simulink model "full_system_boat"  (R2025b)
settings: Solver=FixedStepAuto  StartTime=0.0  StopTime=90  RelTol=1e-3  EnableMultiTasking=on
libraries: arduinolib x7, arduinowifilib x6, dspnetwork x3
settings Model: ExtModeTrigDuration=2  Creator=M  LastModifiedBy=M
settings SolverCC: AutoInsertRateTranBlk=on
settings OptimizationCC: EnhancedBackFolding=on  PassReuseOutputArgsAs=Individual arguments  ZeroExternalMemoryAtStartup=off  ZeroInternalMemoryAtStartup=off  MaxStackSize=64  OptimizeBlockOrder=speed  DifferentSizesBufferReuse=on  OptimizationCustomize=off  EfficientTunableParamExpr=on
settings DebuggingCC: ParameterTunabilityLossMsg=error
settings HardwareCC: ProdBitPerPointer=32.0  ProdBitPerSizeT=32.0  ProdBitPerPtrDiffT=32.0  ProdLargestAtomicInteger=Long  ProdLargestAtomicFloat=Double  ProdWordSize=32.0  ProdHWDeviceType=ARM Compatible->ARM Cortex  UseEmbeddedCoderFeatures=off  UseSimulinkCoderFeatures=off
settings SFSimCC: MATLABDynamicMemAlloc=off
settings RTWCC: SystemTargetFile=ert.tlc  HardwareBoard=ESP32-WROOM (Arduino Compatible)  TLCOptions="-aInlineSetEventsForThisBaseRateFcn=TLC_FALSE -aSuppressMultiTaskScheduler=TLC_FALSE  -aRateBasedStepFcn=0"  TemplateMakefile=ert_default_tmf  Toolchain=ESP32  BuildConfiguration=Faster Runs  Description=Embedded Coder
settings CodeAppCC: ForceParamTrailComments=on  IgnoreCustomStorageClasses=off  OperatorAnnotations=on  SimulinkDataObjDesc=on  SFDataObjDesc=on  MangleLength=10.0  InsertBlockDesc=on
settings ERTTargetCC: ExtModeTransport=3.0  ExtModeStaticAlloc=on  ExtModeAutomaticAllocSize=off  ExtModeStaticAllocSize=65536.0  ExtModeMexFile=ext_xcp  ExtModeIntrfLevel=Level2 - Open  InlinedParameterPlacement=Hierarchical  SupportContinuousTime=on  SupportNonInlinedSFcns=on  SupportVariableSizeSignals=on

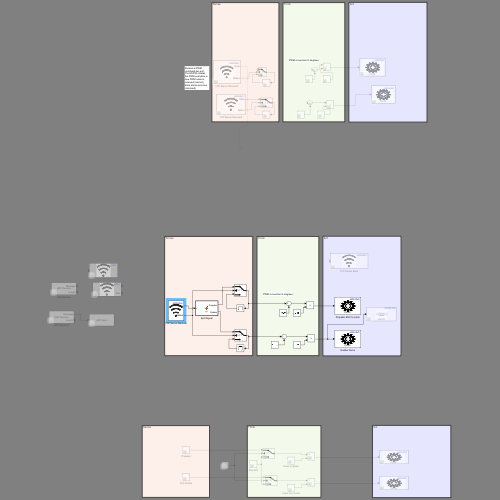
[thumbnail: Simulink's stored preview of the top-level diagram]
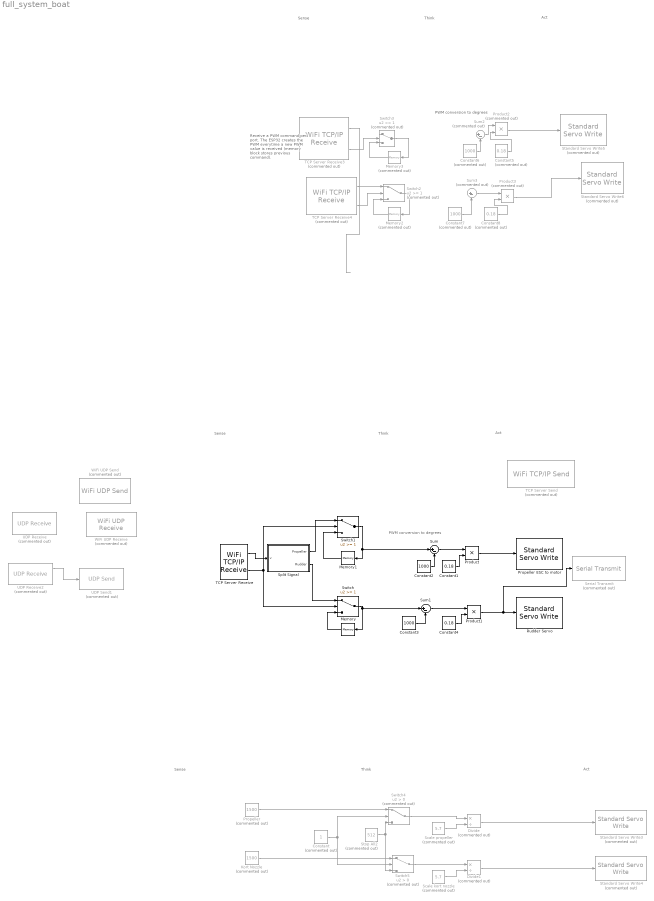
== system full_system_boat ==
  note: Think
  note: PWM conversion to degrees
  note: Sense
  note: Act
  note: Sense
  note: Think
  note: Act
  note: Sense
  note: Receive a PWM command per port. The ESP32 creates the PWM everytime a new PWM value is received (memory block stores previous command).
  note: Act
  note: PWM conversion to degrees
  note: Think
  Constant : Constant  Commented=on  OutDataTypeStr=double
  Constant1 : Constant  Value=0.18  OutDataTypeStr=single
  Constant2 : Constant  Value=1000  OutDataTypeStr=single
  Constant3 : Constant  Value=1000  OutDataTypeStr=single
  Constant4 : Constant  Value=0.18  OutDataTypeStr=single
  Constant5 : Constant  Commented=on  Value=0.18  OutDataTypeStr=single
  Constant6 : Constant  Commented=on  Value=1000  OutDataTypeStr=single
  Constant7 : Constant  Commented=on  Value=1000  OutDataTypeStr=single
  Constant8 : Constant  Commented=on  Value=0.18  OutDataTypeStr=single
  Divide : Product  Commented=on  Inputs=*/
  Divide1 : Product  Commented=on  Inputs=*/
  Kort Nozzle : Constant  Commented=on  Value=1500  OutDataTypeStr=double
  Memory : Memory  InitialCondition=1500
  Memory1 : Memory  InitialCondition=1500
  Memory2 : Memory  Commented=on  InitialCondition=1500
  Memory3 : Memory  Commented=on  InitialCondition=1500
  Product : Product  OutDataTypeStr=single  RndMeth=Nearest
  Product1 : Product  OutDataTypeStr=single  RndMeth=Nearest
  Product2 : Product  Commented=on  OutDataTypeStr=single  RndMeth=Nearest
  Product3 : Product  Commented=on  OutDataTypeStr=single  RndMeth=Nearest
  Propeller : Constant  Commented=on  Value=1500  OutDataTypeStr=double
  Propeller ESC to motor : arduinolib/Standard Servo Write  pinNumber=26  ServoIndex=0  blockPlatform=ESP32
  Rudder Servo : arduinolib/Standard Servo Write  pinNumber=25  ServoIndex=1  blockPlatform=ESP32
  Scale kort nozzle : Constant  Commented=on  Value=5.7
  Scale propeller : Constant  Commented=on  Value=5.7
  Serial Transmit : arduinolib/Serial Transmit  Commented=on  portNumber=0  sendmode=println  label=prop=  sendformat=Decimal  floatprecision=1  header=[]  terminator=[]  blockPlatform=ARDUINO
  Split Signal : MATLAB Function  TreatAsAtomicUnit=on
  Standard Servo Write3 : arduinolib/Standard Servo Write  Commented=on  pinNumber=26  ServoIndex=0  blockPlatform=ESP32
  Standard Servo Write4 : arduinolib/Standard Servo Write  Commented=on  pinNumber=25  ServoIndex=1  blockPlatform=ESP32
  Standard Servo Write5 : arduinolib/Standard Servo Write  Commented=on  pinNumber=26  ServoIndex=0  blockPlatform=ESP32
  Standard Servo Write6 : arduinolib/Standard Servo Write  Commented=on  pinNumber=25  ServoIndex=0  blockPlatform=ESP32
  Stop All2 : Constant  Commented=on  Value=512  OutDataTypeStr=double
  Sum : Sum  Inputs=|+-  OutDataTypeStr=single  RndMeth=Nearest
  Sum1 : Sum  Inputs=|+-  OutDataTypeStr=single  RndMeth=Nearest
  Sum2 : Sum  Commented=on  Inputs=|+-  OutDataTypeStr=single  RndMeth=Nearest
  Sum3 : Sum  Commented=on  Inputs=|+-  OutDataTypeStr=single  RndMeth=Nearest
  Switch : Switch  Threshold=1  RndMeth=Nearest  SaturateOnIntegerOverflow=off  InputSameDT=off
  Switch1 : Switch  Threshold=1  RndMeth=Nearest  SaturateOnIntegerOverflow=off  InputSameDT=off
  Switch2 : Switch  Commented=on  Threshold=1  RndMeth=Nearest  SaturateOnIntegerOverflow=off  InputSameDT=off
  Switch3 : Switch  Commented=on  Threshold=1  RndMeth=Nearest  SaturateOnIntegerOverflow=off  InputSameDT=off
  Switch4 : Switch  Commented=on  Criteria=u2 > Threshold  RndMeth=Nearest  SaturateOnIntegerOverflow=off  InputSameDT=off
  Switch5 : Switch  Commented=on  Criteria=u2 > Threshold  SaturateOnIntegerOverflow=off  InputSameDT=off
  TCP Server Receive : arduinowifilib/WiFi TCP//IP Receive  Mode_=Server  serverport=2000  RemoteAddr_=192.168.137.1  RemoteServerPort_=10000  DataType_=single  DataSize_=2  SampleTime_=0.02  remoteipoctet1=192  remoteipoctet2=168  remoteipoctet3=137  remoteipoctet4=1  wifiTCPServerIndex=0  wifiTCPClientIndex=0  blockPlatform=ARDUINO  isARMArch=false  BlockingMode_=off  BlockTimeout_=0.03
  TCP Server Receive3 : arduinowifilib/WiFi TCP//IP Receive  Commented=on  Mode_=Server  serverport=20001  RemoteAddr_=192.168.137.1  RemoteServerPort_=10000  DataType_=uint8  DataSize_=2  SampleTime_=0.02  remoteipoctet1=192  remoteipoctet2=168  remoteipoctet3=137  remoteipoctet4=1  wifiTCPServerIndex=0  wifiTCPClientIndex=0  blockPlatform=ARDUINO  isARMArch=false  BlockingMode_=off  BlockTimeout_=0.03
  TCP Server Receive4 : arduinowifilib/WiFi TCP//IP Receive  Commented=on  Mode_=Server  serverport=20002  RemoteAddr_=192.168.137.1  RemoteServerPort_=10000  DataType_=single  DataSize_=1  SampleTime_=0.02  remoteipoctet1=192  remoteipoctet2=168  remoteipoctet3=137  remoteipoctet4=1  wifiTCPServerIndex=1  wifiTCPClientIndex=0  blockPlatform=ARDUINO  isARMArch=false  BlockingMode_=off  BlockTimeout_=0.03
  TCP Server Send : arduinowifilib/WiFi TCP//IP Send  Commented=on  Mode_=Server  serverport=20001  RemoteAddr_=192.168.137.1  RemoteServerPort_=10000  remoteipoctet1=192  remoteipoctet2=168  remoteipoctet3=137  remoteipoctet4=1  wifiTCPServerIndex=0  wifiTCPClientIndex=0  blockPlatform=ARDUINO  isARMArch=false
  UDP Receive : dspnetwork/UDP Receive  Commented=on  localURL='0.0.0.0'  localPort=20000  remoteURL='192.168.137.1'  remotePort=-1  recvBufferSize=32  dims=32  signalDatatype=single  isComplex=off  isVarSize=off  showBlockingTime=off  blockingTime=0  sampletime=0.02  blockPlatform=[]
      settings: LibrarySourceBlock=dspsrcs4/UDP Receive
  UDP Receive2 : dspnetwork/UDP Receive  Commented=on  localURL='0.0.0.0'  localPort=20000  remoteURL='192.168.137.1'  remotePort=-1  recvBufferSize=8192  dims=255  signalDatatype=uint8  isComplex=off  isVarSize=off  showBlockingTime=off  blockingTime=0  sampletime=0.02  blockPlatform=[]
      settings: LibrarySourceBlock=dspsrcs4/UDP Receive
  UDP Send1 : dspnetwork/UDP Send  Commented=on  remoteURL='192.168.137.1'  remotePort=10000  localURL='0.0.0.0'  localPortSource=Specify via dialog  localPort=20000  sendBufferSize=8192  sampletime=-1  blockPlatform=[]  separateLengthPort=0
      settings: LibrarySourceBlock=dspsnks4/UDP Send
  WiFi UDP Receive : arduinowifilib/WiFi UDP Receive  Commented=on  localport=20000  DataType=single  DataLength=1  SampleTime_=-1  wifiUDPIndex=0  blockPlatform=ARDUINO  isARMArch=false
  WiFi UDP Send : arduinowifilib/WiFi UDP Send  Commented=on  remoteIPOctetString=192.168.137.1  remoteport=10000  localport=20000  remoteipoctet1=192  remoteipoctet2=168  remoteipoctet3=137  remoteipoctet4=1  wifiUDPIndex=0  blockPlatform=ARDUINO  isARMArch=false
  wires:
  Sum1/1 -> Product1/1
  UDP Receive2/1 -> UDP Send1/1
  Stop All2/1 -> Switch5/3, Switch4/3
  Scale kort nozzle/1 -> Divide1/2
  Divide/1 -> Standard Servo Write3/1
  Constant/1 -> Switch4/2, Switch5/2
  Divide1/1 -> Standard Servo Write4/1
  Switch4/1 -> Divide/1
  Scale propeller/1 -> Divide/2
  Switch5/1 -> Divide1/1
  Propeller/1 -> Switch4/1
  Kort Nozzle/1 -> Switch5/1
  Constant2/1 -> Sum/2
  Sum/1 -> Product/1
  Constant1/1 -> Product/2
  Constant4/1 -> Product1/2
  TCP Server Receive/2 -> Switch/2, Switch1/2
  Split Signal/2(Rudder) -> Switch/1
  Switch/1 -> Sum1/1, Memory/1
  Memory/1 -> Switch/3
  Memory1/1 -> Switch1/3
  Constant3/1 -> Sum1/2
  Switch1/1 -> Sum/1, Memory1/1
  TCP Server Receive4/2 -> Switch2/2
  Constant7/1 -> Sum3/2
  Constant8/1 -> Product3/2
  Product2/1 -> Standard Servo Write5/1
  Memory2/1 -> Switch2/3
  Sum3/1 -> Product3/1
  Product3/1 -> Standard Servo Write6/1
  Switch3/1 -> Memory3/1
  Sum2/1 -> Product2/1
  Constant6/1 -> Sum2/2
  Switch2/1 -> Memory2/1
  Memory3/1 -> Switch3/3
  TCP Server Receive3/2 -> Switch3/2
  TCP Server Receive3/1 -> ?
  Constant5/1 -> Product2/2
  TCP Server Receive4/1 -> Switch2/1
  TCP Server Receive/1 -> Split Signal/1(v)
  Split Signal/1(Propeller) -> Switch1/1
  Product/1 -> Propeller ESC to motor/1
  Product1/1 -> Serial Transmit/1, Rudder Servo/1

== matlab function full_system_boat/Split Signal ==
  data: v input; Propeller output; Rudder output
function [Propeller,Rudder] = fcn(v)

Propeller = v(1);
Rudder = v(2);

end
